simulink model "Encoder_reader_simulink"  (R2025a)
settings: Solver=FixedStepAuto  StartTime=0.0  StopTime=inf  FixedStep=0.1  RelTol=1e-3  EnableMultiTasking=on
libraries: stm32f4xxblockslib x9, stm32g4xxblockslib x4
settings Model: STM32="{\"EncoderBlockForG4\":[{\"ID\":\"untitled:1\"},{\"ID\":\"Lab3_Encoder:1\"},{\"ID\":\"Encoder_reader_simulink:1\"},{\"ID\":\"Encoder_reader_simulink:83\"},{\"ID\":\"Encoder_reader_simulink:126\"},{\"ID\":\"Encoder_reader_simulink:148\"}],\"DigitalPortRead\":[{\"ID\":\"Encoder_reader_simulink:48\"},{\"ID\":\"Encoder_reader_simulink:49\"},{\"ID\":\"Encoder_reader_simulink:52\"},{\"ID\":\"Encoder_reader_simulink:80\"},{\"ID\":\"Encoder_reader_simulink:112\"},{\"ID\":\"Encoder_reader_simulink:120\"},{\"ID\":\"Encoder_reader_simulink:134\"},{\"ID\":\"Encoder_reader_simulink:136\"},{\"ID\":\"Encoder_reader_simulink:142\"}]}"  Creator=User  LastModifiedBy=putth
settings SolverCC: AutoInsertRateTranBlk=on
settings OptimizationCC: DefaultParameterBehavior=Inlined  EnhancedBackFolding=on  PassReuseOutputArgsAs=Individual arguments  ZeroExternalMemoryAtStartup=off  ZeroInternalMemoryAtStartup=off  MaxStackSize=512  OptimizeBlockOrder=speed  DifferentSizesBufferReuse=on  OptimizationCustomize=off  EfficientTunableParamExpr=on
settings DebuggingCC: ParameterTunabilityLossMsg=error
settings HardwareCC: ProdBitPerPointer=32.0  ProdBitPerSizeT=32.0  ProdBitPerPtrDiffT=32.0  ProdLargestAtomicInteger=Long  ProdLargestAtomicFloat=Double  ProdWordSize=32.0  ProdLongLongMode=on  ProdHWDeviceType=ARM Compatible->ARM Cortex-M
settings SFSimCC: MATLABDynamicMemAlloc=off
settings RTWCC: SystemTargetFile=ert.tlc  HardwareBoard=STM32G4xx Based  TemplateMakefile=ert_default_tmf  Toolchain=GNU Tools for ARM Embedded Processors  Description=Embedded Coder
settings CodeAppCC: ForceParamTrailComments=on  IgnoreCustomStorageClasses=off  OperatorAnnotations=on  SimulinkDataObjDesc=on  SFDataObjDesc=on  InsertBlockDesc=on
settings ERTTargetCC: ExtModeTransport=3.0  ExtModeStaticAllocSize=2048.0  TargetLangStandard=C99 (ISO)  CodeReplacementLibrary=ARM Cortex-M  SupportContinuousTime=on

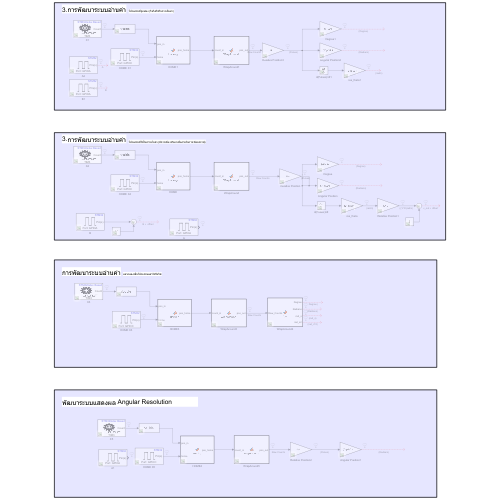
[thumbnail: Simulink's stored preview of the top-level diagram]
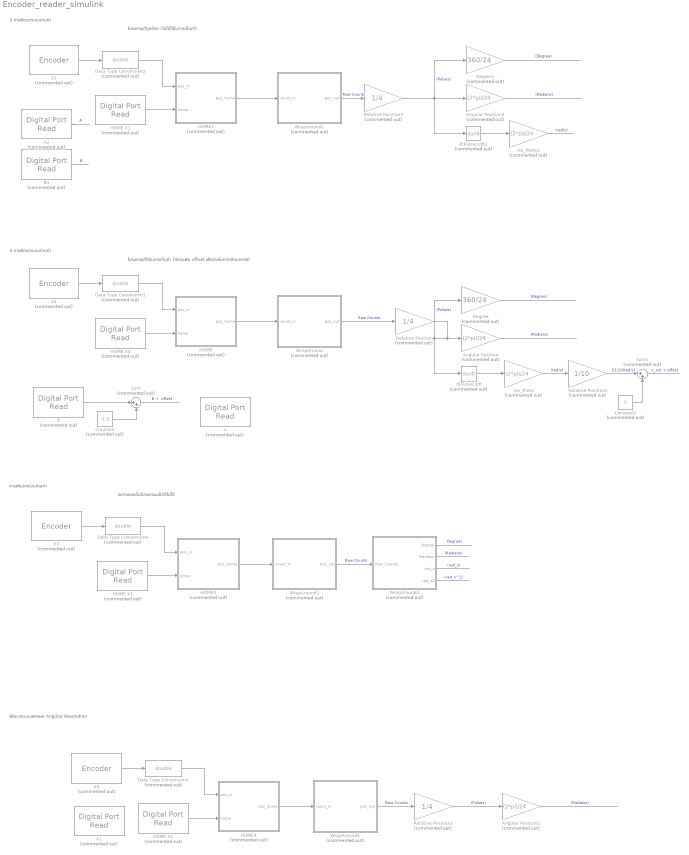
== system Encoder_reader_simulink ==
  note: 3.การพัฒนาระบบอ่านค่า
  note: การพัฒนาระบบอ่านค่า
  note: พัฒนาระบบแสดงผล Angular Resolution
  note: อยากลองเป็นโปรแกรมแล้วใช้ไม่ได้
  note: 3.การพัฒนาระบบอ่านค่า
  note: โปรแกรมที่ถูกต้อง (ไม่ได้ใช้ในการเก็บค่า)
  note: โปรแกรมที่ใช้ในการเก็บค่า (มีการเพิ่ม offset เพื่อง่ายในการเทียบกราฟ)
  A : stm32f4xxblockslib/Digital Port Read  Commented=on  PortName=GPIOA  PinNumber=[6]  ReadOperation=on  IOAsArray=on  SampleTime=0.1  EnableSimPort=off  hoistedMaskSrc=ECSoC/ECSimCodegen/Digital Port Read
      settings: LibrarySourceBlock=stm32g4xxblockslib/Digital Port Read
  A1 : stm32f4xxblockslib/Digital Port Read  Commented=on  PortName=GPIOA  PinNumber=[6]  ReadOperation=on  IOAsArray=on  SampleTime=0.1  EnableSimPort=off  hoistedMaskSrc=ECSoC/ECSimCodegen/Digital Port Read
      settings: LibrarySourceBlock=stm32g4xxblockslib/Digital Port Read
  A2 : stm32f4xxblockslib/Digital Port Read  Commented=on  PortName=GPIOA  PinNumber=[6]  ReadOperation=on  IOAsArray=on  SampleTime=0.1  EnableSimPort=off  hoistedMaskSrc=ECSoC/ECSimCodegen/Digital Port Read
      settings: LibrarySourceBlock=stm32g4xxblockslib/Digital Port Read
  Angular Position : Gain  Commented=on  Gain=(2*pi)/24
  Angular Position1 : Gain  Commented=on  Gain=(2*pi)/24
  Angular Position2 : Gain  Commented=on  Gain=(2*pi)/24
  B : stm32f4xxblockslib/Digital Port Read  Commented=on  PortName=GPIOA  PinNumber=[4]  ReadOperation=on  IOAsArray=on  SampleTime=0.1  EnableSimPort=off  hoistedMaskSrc=ECSoC/ECSimCodegen/Digital Port Read
      settings: LibrarySourceBlock=stm32g4xxblockslib/Digital Port Read
  B1 : stm32f4xxblockslib/Digital Port Read  Commented=on  PortName=GPIOA  PinNumber=[4]  ReadOperation=on  IOAsArray=on  SampleTime=0.1  EnableSimPort=off  hoistedMaskSrc=ECSoC/ECSimCodegen/Digital Port Read
      settings: LibrarySourceBlock=stm32g4xxblockslib/Digital Port Read
  Constant : Constant  Commented=on  Value=-1.5
  Constant1 : Constant  Commented=on  Value=5
  Data Type Conversion{1..2,4..5} (4 alike) : DataTypeConversion  Commented=on  OutDataTypeStr=double  SaturateOnIntegerOverflow=off  RndMeth=Floor
  Degree : Gain  Commented=on  Gain=360/24
  Degree1 : Gain  Commented=on  Gain=360/24
  HOME : MATLAB Function  Commented=on  TreatAsAtomicUnit=on
  HOME X{1,3..5} (4 alike) : stm32f4xxblockslib/Digital Port Read  Commented=on  PortName=GPIOC  PinNumber=[13]  ReadOperation=on  IOAsArray=on  SampleTime=0.1  EnableSimPort=off  hoistedMaskSrc=ECSoC/ECSimCodegen/Digital Port Read
      settings: LibrarySourceBlock=stm32g4xxblockslib/Digital Port Read
  HOME1 : MATLAB Function  Commented=on  TreatAsAtomicUnit=on
  HOME3 : MATLAB Function  Commented=on  TreatAsAtomicUnit=on
  HOME4 : MATLAB Function  Commented=on  TreatAsAtomicUnit=on
  Relative Position : Gain  Commented=on  Gain=1/4
  Relative Position1 : Gain  Commented=on  Gain=1/10
  Relative Position2 : Gain  Commented=on  Gain=1/4
  Relative Position3 : Gain  Commented=on  Gain=1/4
  Sum : Sum  Commented=on  Inputs=|++
  Sum1 : Sum  Commented=on  Inputs=|++
  WrapAround : MATLAB Function  Commented=on  TreatAsAtomicUnit=on
  WrapAround1 : MATLAB Function  Commented=on  TreatAsAtomicUnit=on
  WrapAround3 : MATLAB Function  Commented=on  TreatAsAtomicUnit=on
  WrapAround4 : MATLAB Function  Commented=on  TreatAsAtomicUnit=on
  WrapAround5 : MATLAB Function  Commented=on  TreatAsAtomicUnit=on
  X{1,3..5} (4 alike) : stm32g4xxblockslib/Encoder  Commented=on  TimerModule=TIM3  EnableResetInput=off  OutputCountAfterFirstIndex=off  OutputValidIndex=off  OutputDirection=off  OutputStatus=off  SampleTime=-1
  d(Pulses)/dt : Derivative  Commented=on
  d(Pulses)/dt1 : Derivative  Commented=on
  res_theta : Gain  Commented=on  Gain=(2*pi)/24
  res_theta1 : Gain  Commented=on  Gain=(2*pi)/24
  wires:
  X4/1 -> Data Type Conversion1/1
  Data Type Conversion1/1 -> HOME/1(pos_in)
  WrapAround/1(pos_out) -> Relative Position/1  "Raw Counts"
  HOME/1(pos_home) -> WrapAround/1(count_in)
  HOME X4/1 -> HOME/2(home)
  Relative Position/1 -> Degree/1, d(Pulses)/dt/1, Angular Position/1  "(Pulses)"
  Angular Position/1 -> ?  "(Radians)"
  d(Pulses)/dt/1 -> res_theta/1
  res_theta/1 -> Relative Position1/1  "(rad/s)"
  Degree/1 -> ?  "(Degree)"
  HOME3/1(pos_home) -> WrapAround3/1(count_in)
  WrapAround3/1(pos_out) -> WrapAround4/1(Raw_Counts)  "Raw Counts"
  Data Type Conversion4/1 -> HOME3/1(pos_in)
  HOME X3/1 -> HOME3/2(home)
  X3/1 -> Data Type Conversion4/1
  WrapAround4/1(Degree) -> ?  "Degree)"
  WrapAround4/2(Radians) -> ?  "(Radians)"
  WrapAround4/3(rad_s) -> ?  "(rad_s)"
  WrapAround4/4(rad_s2) -> ?  "(rad_s^2)"
  B/1 -> Sum/1
  Constant/1 -> Sum/2
  Sum/1 -> ?  "B +  offset"
  Relative Position1/1 -> Sum1/1  "((1/10)rad/s)"
  Constant1/1 -> Sum1/2
  Sum1/1 -> ?  "v_out + offset"
  Angular Position1/1 -> ?  "(Radians)"
  HOME X5/1 -> HOME4/2(home)
  Relative Position2/1 -> Angular Position1/1  "(Pulses)"
  HOME4/1(pos_home) -> WrapAround5/1(count_in)
  X5/1 -> Data Type Conversion5/1
  WrapAround5/1(pos_out) -> Relative Position2/1  "Raw Counts"
  Data Type Conversion5/1 -> HOME4/1(pos_in)
  Angular Position2/1 -> ?  "(Radians)"
  Degree1/1 -> ?  "(Degree)"
  X1/1 -> Data Type Conversion2/1
  HOME X1/1 -> HOME1/2(home)
  B1/1 -> ?  "B"
  HOME1/1(pos_home) -> WrapAround1/1(count_in)
  res_theta1/1 -> ?  "(rad/s)"
  Relative Position3/1 -> d(Pulses)/dt1/1, Angular Position2/1, Degree1/1  "(Pulses)"
  Data Type Conversion2/1 -> HOME1/1(pos_in)
  d(Pulses)/dt1/1 -> res_theta1/1
  WrapAround1/1(pos_out) -> Relative Position3/1  "Raw Counts"
  A2/1 -> ?  "A"

== matlab function Encoder_reader_simulink/HOME1 ==
  data: pos_in input; pos_home output; home input
function pos_home = Homing(pos_in, home)
%#codegen
persistent offset init

if isempty(init)
    offset = 0;
    init = true;
end
    
if home == 1
    offset = pos_in; % จดจำค่าปัจจุบันเป็นจุดอ้างอิง
end

pos_home = pos_in - offset; % หักออกให้ตำแหน่งปัจจุบันกลายเป็นศูนย์
end

== matlab function Encoder_reader_simulink/WrapAround ==
  data: count_in input; pos_out output
function pos_out = WrapAround(count_in)
%#codegen

% --- ค่าคงที่ ---
MAX_COUNT = 61439;   % จาก IOC Counter Period
HALF_COUNT = MAX_COUNT / 2;

% --- ตัวแปรคงอยู่ข้ามรอบ ---
persistent old_count;
persistent total_count;

if isempty(old_count)
    old_count = 0;
    total_count = 0;
end

% --- คำนวณการเปลี่ยนแปลง ---
diff = count_in - old_count;

% --- ตรวจจับการข้ามรอบ (Wrap-around) ---
if diff > HALF_COUNT
    % หมุนย้อนกลับจาก 0 -> MAX
    diff = diff - (MAX_COUNT + 1);
elseif diff < -HALF_COUNT
    % หมุนต่อจาก MAX -> 0
    diff = diff + (MAX_COUNT + 1);
end

% --- รวมค่าการหมุนทั้งหมด ---
total_count = total_count + diff;

% --- ส่งค่าออก (ตำแหน่งต่อเนื่อง) ---
pos_out = total_count;

% --- อัปเดตค่าเดิม ---
old_count = count_in;

== matlab function Encoder_reader_simulink/WrapAround1 ==
  data: count_in input; pos_out output
function pos_out = WrapAround(count_in)
%#codegen

% --- ค่าคงที่ ---
MAX_COUNT = 61439;   % จาก IOC Counter Period
HALF_COUNT = MAX_COUNT / 2;

% --- ตัวแปรคงอยู่ข้ามรอบ ---
persistent old_count;
persistent total_count;

if isempty(old_count)
    old_count = 0;
    total_count = 0;
end

% --- คำนวณการเปลี่ยนแปลง ---
diff = count_in - old_count;

% --- ตรวจจับการข้ามรอบ (Wrap-around) ---
if diff > HALF_COUNT
    % หมุนย้อนกลับจาก 0 -> MAX
    diff = diff - (MAX_COUNT + 1);
elseif diff < -HALF_COUNT
    % หมุนต่อจาก MAX -> 0
    diff = diff + (MAX_COUNT + 1);
end

% --- รวมค่าการหมุนทั้งหมด ---
total_count = total_count + diff;

% --- ส่งค่าออก (ตำแหน่งต่อเนื่อง) ---
pos_out = total_count;

% --- อัปเดตค่าเดิม ---
old_count = count_in;

== matlab function Encoder_reader_simulink/HOME ==
  data: pos_in input; pos_home output; home input
function pos_home = Homing(pos_in, home)
%#codegen
persistent offset init

if isempty(init)
    offset = 0;
    init = true;
end
    
if home == 1
    offset = pos_in; % จดจำค่าปัจจุบันเป็นจุดอ้างอิง
end

pos_home = pos_in - offset; % หักออกให้ตำแหน่งปัจจุบันกลายเป็นศูนย์
end

== matlab function Encoder_reader_simulink/HOME3 ==
  data: pos_in input; pos_home output; home input
function pos_home = Homing(pos_in, home)
%#codegen
persistent offset init

if isempty(init)
    offset = 0;
    init = true;
end
    
if home == 1
    offset = pos_in; % จดจำค่าปัจจุบันเป็นจุดอ้างอิง
end

pos_home = pos_in - offset; % หักออกให้ตำแหน่งปัจจุบันกลายเป็นศูนย์
end

== matlab function Encoder_reader_simulink/WrapAround3 ==
  data: count_in input; pos_out output
function pos_out = WrapAround(count_in)
%#codegen

% --- ค่าคงที่ ---
MAX_COUNT = 61439;   % จาก IOC Counter Period
HALF_COUNT = MAX_COUNT / 2;

% --- ตัวแปรคงอยู่ข้ามรอบ ---
persistent old_count;
persistent total_count;

if isempty(old_count)
    old_count = 0;
    total_count = 0;
end

% --- คำนวณการเปลี่ยนแปลง ---
diff = count_in - old_count;

% --- ตรวจจับการข้ามรอบ (Wrap-around) ---
if diff > HALF_COUNT
    % หมุนย้อนกลับจาก 0 -> MAX
    diff = diff - (MAX_COUNT + 1);
elseif diff < -HALF_COUNT
    % หมุนต่อจาก MAX -> 0
    diff = diff + (MAX_COUNT + 1);
end

% --- รวมค่าการหมุนทั้งหมด ---
total_count = total_count + diff;

% --- ส่งค่าออก (ตำแหน่งต่อเนื่อง) ---
pos_out = total_count;

% --- อัปเดตค่าเดิม ---
old_count = count_in;

== matlab function Encoder_reader_simulink/WrapAround4 ==
  data: Raw_Counts input; Degree output; Radians output; rad_s output; rad_s2 output
function [Degree, Radians, rad_s, rad_s2] = fun(Raw_Counts)

x = 4;
Pulse = 24;
Ts = 0.01;  % กำหนด sampling time ของ encoder (หน่วยวินาที)
restheta = (2*pi)/Pulse;
Relativ_Position = Raw_Counts / x;

Degree  = Relativ_Position * (360 / Pulse);
Radians = Relativ_Position * (2*pi / Pulse);

% --- คำนวณ angular velocity ---
rad_s_temp = [0; diff(Raw_Counts)] / Ts;  % หารด้วยเวลา
rad_s  = restheta * rad_s_temp;

% --- คำนวณ angular acceleration ---
rad_s2_temp = [0; diff(rad_s)] / Ts;
rad_s2 = rad_s2_temp;
end

== matlab function Encoder_reader_simulink/HOME4 ==
  data: pos_in input; pos_home output; home input
function pos_home = Homing(pos_in, home)
%#codegen
persistent offset init

if isempty(init)
    offset = 0;
    init = true;
end
    
if home == 1
    offset = pos_in; % จดจำค่าปัจจุบันเป็นจุดอ้างอิง
end

pos_home = pos_in - offset; % หักออกให้ตำแหน่งปัจจุบันกลายเป็นศูนย์
end

== matlab function Encoder_reader_simulink/WrapAround5 ==
  data: count_in input; pos_out output
function pos_out = WrapAround(count_in)
%#codegen

% --- ค่าคงที่ ---
MAX_COUNT = 61439;   % จาก IOC Counter Period
HALF_COUNT = MAX_COUNT / 2;

% --- ตัวแปรคงอยู่ข้ามรอบ ---
persistent old_count;
persistent total_count;

if isempty(old_count)
    old_count = 0;
    total_count = 0;
end

% --- คำนวณการเปลี่ยนแปลง ---
diff = count_in - old_count;

% --- ตรวจจับการข้ามรอบ (Wrap-around) ---
if diff > HALF_COUNT
    % หมุนย้อนกลับจาก 0 -> MAX
    diff = diff - (MAX_COUNT + 1);
elseif diff < -HALF_COUNT
    % หมุนต่อจาก MAX -> 0
    diff = diff + (MAX_COUNT + 1);
end

% --- รวมค่าการหมุนทั้งหมด ---
total_count = total_count + diff;

% --- ส่งค่าออก (ตำแหน่งต่อเนื่อง) ---
pos_out = total_count;

% --- อัปเดตค่าเดิม ---
old_count = count_in;
